simulink model "Copter_Plane_h2g_4_and_1_out"  (R2020a)
settings: Solver=ode1  StartTime=0.0  StopTime=1  FixedStep=dt  RelTol=1e-3
values from neighbouring files (symbols this model uses):
  center_WP = [40,100]*1e7    [Compter_Plane_inint_m_V10.m]    (also in Compter_Plane_inint_m_fs_form_V1031.m; Compter_Plane_inint_m_fs_form_V1032.m; Compter_Plane_inint_m_fs_form_V10321.m; Compter_Plane_inint_m_fs_form_V10321_4a1.m)
  Euler = [5/HD 5/HD 30/HD]    [Compter_Plane_inint_m_V10g.m]
  GRAVITY_MSS = 9.80665    [Compter_Plane_inint_m_V10.m]    (also in Compter_Plane_inint_m_V10g.m; Compter_Plane_inint_m_fs_form_V1031.m; Compter_Plane_inint_m_fs_form_V1032.m; Compter_Plane_inint_m_fs_form_V10321.m)
  gyro_x = 0    [Compter_Plane_inint_m_V10.m]    (also in Compter_Plane_inint_m_fs_form_V1031.m; Compter_Plane_inint_m_fs_form_V1032.m; Compter_Plane_inint_m_fs_form_V10321.m; Compter_Plane_inint_m_fs_form_V10321_4a1.m)
  gyro_y = 0/HD    (= 0)    [Compter_Plane_inint_m_V10.m]    (also in Compter_Plane_inint_m_fs_form_V1031.m; Compter_Plane_inint_m_fs_form_V1032.m; Compter_Plane_inint_m_fs_form_V10321.m; Compter_Plane_inint_m_fs_form_V10321_4a1.m)
  gyro_z = 0    [Compter_Plane_inint_m_V10.m]    (also in Compter_Plane_inint_m_fs_form_V1031.m; Compter_Plane_inint_m_fs_form_V1032.m; Compter_Plane_inint_m_fs_form_V10321.m; Compter_Plane_inint_m_fs_form_V10321_4a1.m)
  HD = 180/pi    (= 57.2957795131)    [Compter_Plane_inint_m_V10.m]    (also in Compter_Plane_inint_m_V10g.m; Compter_Plane_inint_m_fs_form_V1031.m; Compter_Plane_inint_m_fs_form_V1032.m; Compter_Plane_inint_m_fs_form_V10321.m)
  J = J_V10    [Compter_Plane_inint_m_V10.m]    (also in Compter_Plane_inint_m_V10g.m)
  Kd = Ku*Luy/Ldy    (= 18.9029535865)    [Compter_Plane_inint_m_V10.m]    (also in Compter_Plane_inint_m_fs_form_V1031.m; Compter_Plane_inint_m_fs_form_V1032.m; Compter_Plane_inint_m_fs_form_V10321.m; Compter_Plane_inint_m_fs_form_V10321_4a1.m)
  Ku = 32    [Compter_Plane_inint_m_V10.m]    (also in Compter_Plane_inint_m_fs_form_V1031.m; Compter_Plane_inint_m_fs_form_V1032.m; Compter_Plane_inint_m_fs_form_V10321.m; Compter_Plane_inint_m_fs_form_V10321_4a1.m)
  Ld = hypot(Ldx,Ldy)    [Compter_Plane_inint_m_V10.m]    (also in Compter_Plane_inint_m_fs_form_V1031.m; Compter_Plane_inint_m_fs_form_V1032.m; Compter_Plane_inint_m_fs_form_V10321.m; Compter_Plane_inint_m_fs_form_V10321_4a1.m)
  Ldx = 205/1000    (= 0.205)    [Compter_Plane_inint_m_V10.m]    (also in Compter_Plane_inint_m_fs_form_V1031.m; Compter_Plane_inint_m_fs_form_V1032.m; Compter_Plane_inint_m_fs_form_V10321.m; Compter_Plane_inint_m_fs_form_V10321_4a1.m)
  Ldy = 355.5/1000    (= 0.3555)    [Compter_Plane_inint_m_V10.m]    (also in Compter_Plane_inint_m_fs_form_V1031.m; Compter_Plane_inint_m_fs_form_V1032.m; Compter_Plane_inint_m_fs_form_V10321.m; Compter_Plane_inint_m_fs_form_V10321_4a1.m)
  Lu = hypot(Lux,Luy)    [Compter_Plane_inint_m_V10.m]    (also in Compter_Plane_inint_m_fs_form_V1031.m; Compter_Plane_inint_m_fs_form_V1032.m; Compter_Plane_inint_m_fs_form_V10321.m; Compter_Plane_inint_m_fs_form_V10321_4a1.m)
  Lux = 310/1000    (= 0.31)    [Compter_Plane_inint_m_V10.m]    (also in Compter_Plane_inint_m_fs_form_V1031.m; Compter_Plane_inint_m_fs_form_V1032.m; Compter_Plane_inint_m_fs_form_V10321.m; Compter_Plane_inint_m_fs_form_V10321_4a1.m)
  Luy = 210/1000    (= 0.21)    [Compter_Plane_inint_m_V10.m]    (also in Compter_Plane_inint_m_fs_form_V1031.m; Compter_Plane_inint_m_fs_form_V1032.m; Compter_Plane_inint_m_fs_form_V10321.m; Compter_Plane_inint_m_fs_form_V10321_4a1.m)
  m_kg = m_kg_V10    (= 26)    [Compter_Plane_inint_m_V10.m]    (also in Compter_Plane_inint_m_V10g.m; Compter_Plane_inint_m_fs_form_V1031.m = 5; Compter_Plane_inint_m_fs_form_V1032.m = 5; Compter_Plane_inint_m_fs_form_V10321.m = 5)
  pitch = -40/HD    (= -0.698131700798)    [Compter_Plane_inint_m_V10.m]    (also in Compter_Plane_inint_m_fs_form_V1031.m = 0; Compter_Plane_inint_m_fs_form_V1032.m = 0; Compter_Plane_inint_m_fs_form_V10321.m = 0; Compter_Plane_inint_m_fs_form_V10321_4a1.m = 0)
  pwm_max = 2000    [Compter_Plane_inint_m_V10.m]    (also in Compter_Plane_inint_m_fs_form_V1031.m; Compter_Plane_inint_m_fs_form_V1032.m; Compter_Plane_inint_m_fs_form_V10321.m; Compter_Plane_inint_m_fs_form_V10321_4a1.m)
  pwm_min = 1000    [Compter_Plane_inint_m_V10.m]    (also in Compter_Plane_inint_m_fs_form_V1031.m; Compter_Plane_inint_m_fs_form_V1032.m; Compter_Plane_inint_m_fs_form_V10321.m; Compter_Plane_inint_m_fs_form_V10321_4a1.m)
  Qd = 10    [Compter_Plane_inint_m_V10.m]    (also in Compter_Plane_inint_m_fs_form_V1031.m; Compter_Plane_inint_m_fs_form_V1032.m; Compter_Plane_inint_m_fs_form_V10321.m; Compter_Plane_inint_m_fs_form_V10321_4a1.m)
  Qu = asind(Kd*sind(Qd)*Ld/(Ku*Lu))    [Compter_Plane_inint_m_V10.m]    (also in Compter_Plane_inint_m_fs_form_V1031.m; Compter_Plane_inint_m_fs_form_V1032.m; Compter_Plane_inint_m_fs_form_V10321.m; Compter_Plane_inint_m_fs_form_V10321_4a1.m)
  roll = 10/HD    (= 0.174532925199)    [Compter_Plane_inint_m_V10.m]    (also in Compter_Plane_inint_m_fs_form_V1031.m = 0; Compter_Plane_inint_m_fs_form_V1032.m = 0; Compter_Plane_inint_m_fs_form_V10321.m = 0; Compter_Plane_inint_m_fs_form_V10321_4a1.m = 0)
  vel_desired = [0 0 0]    [Compter_Plane_inint_m_V10.m]    (also in Compter_Plane_inint_m_fs_form_V1031.m; Compter_Plane_inint_m_fs_form_V1032.m; Compter_Plane_inint_m_fs_form_V10321.m; Compter_Plane_inint_m_fs_form_V10321_4a1.m)
  yaw = 0    [Compter_Plane_inint_m_V10.m]    (also in Compter_Plane_inint_m_fs_form_V1031.m; Compter_Plane_inint_m_fs_form_V1032.m; Compter_Plane_inint_m_fs_form_V10321.m; Compter_Plane_inint_m_fs_form_V10321_4a1.m)
undefined symbols (not defined in the file or in its folder): Newton, QLd, QLdx, QLdy, QLu, QLux, QLuy, Raphson
libraries: shared6dofsys x3, sharedutil x1, simulink x1, aerolibasang x1
(part 1 of 3)
settings Model: xpc_rtwmakecfg_data=_xpcnblib_  PauseTimes=2  Creator=a4327  LastModifiedBy=a4327
settings DataIOCC: ReturnWorkspaceOutputs=off
settings OptimizationCC: DefaultParameterBehavior=Inlined  UseDivisionForNetSlopeComputation=on  GainParamInheritBuiltInType=on  UseFloatMulNetSlope=on  InlineInvariantSignals=on  PassReuseOutputArgsAs=Individual arguments  ZeroExternalMemoryAtStartup=off  ZeroInternalMemoryAtStartup=off  NoFixptDivByZeroProtection=on  EfficientFloat2IntCast=on  LifeSpan=1  OptimizeBlockOrder=speed  DifferentSizesBufferReuse=on  EfficientTunableParamExpr=on
settings DebuggingCC: ParameterTunabilityLossMsg=error  ArithmeticOperatorsInVariantConditions=warning
settings HardwareCC: ProdBitPerPointer=32  ProdBitPerSizeT=32  ProdBitPerPtrDiffT=32  ProdLargestAtomicFloat=None  ProdWordSize=32  ProdLongLongMode=on  ProdHWDeviceType=Custom Processor->Custom Processor
settings SFSimCC: MATLABDynamicMemAlloc=off  CustomCodeUndefinedFunction=UseInterfaceOnly
settings RTWCC: SystemTargetFile=ert.tlc  TemplateMakefile=ert_default_tmf  GenerateReport=on  IncludeHyperlinkInReport=on  LaunchReport=on  GenerateTraceInfo=on  GenerateTraceReport=on  GenerateTraceReportSl=on  GenerateTraceReportSf=on  GenerateTraceReportEml=on  GenerateCodeMetricsReport=on
settings CodeAppCC: ForceParamTrailComments=on  IgnoreCustomStorageClasses=off  OperatorAnnotations=on  SimulinkDataObjDesc=on  SFDataObjDesc=on  CustomSymbolStrGlobalVar=rt$N$M  CustomSymbolStrType=$N$M  CustomSymbolStrFcn=$N$M$F  CustomSymbolStrMacro=$N$M  InsertBlockDesc=on
settings ERTTargetCC: TargetLangStandard=C99 (ISO)  GenerateSampleERTMain=on  IncludeMdlTerminateFcn=off  CombineSignalStateStructs=on  MultiInstanceERTCode=on  CodeInterfacePackaging=Reusable function  SupportComplex=off  SupportNonInlinedSFcns=on  InlinedParameterPlacement=NonHierarchical  RootIOFormat=Structure reference  ERTCustomFileTemplate=example_file_process.tlc  ERTFilePackagingFormat=CompactWithDataFile

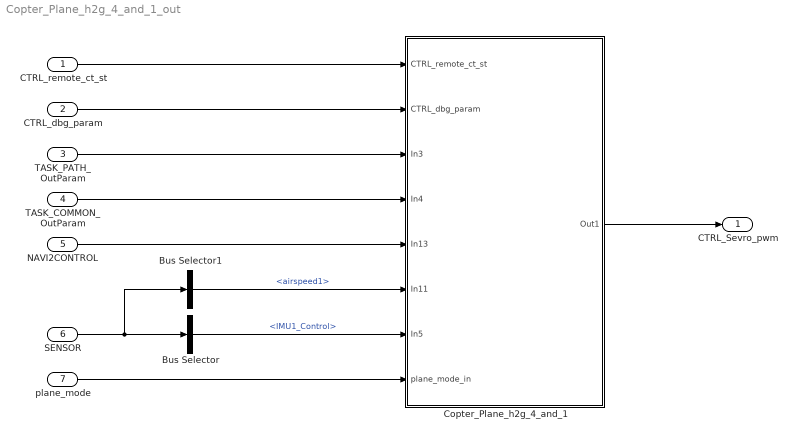
== system Copter_Plane_h2g_4_and_1_out ==
  CTRL_remote_ct_st : Inport  OutDataTypeStr=Bus: BUS_CTRL_remote_ct_st  BusOutputAsStruct=on
  CTRL_dbg_param : Inport  Port=2  OutDataTypeStr=Bus: BUS_CTRL_dbg_param  BusOutputAsStruct=on
  TASK_PATH_OutParam : Inport  Port=3  OutDataTypeStr=Bus: BUS_TASK_PATH_OutParam  BusOutputAsStruct=on
  TASK_COMMON_OutParam : Inport  Port=4  OutDataTypeStr=Bus: BUS_TASK_COMMON_OutParam  BusOutputAsStruct=on
  NAVI2CONTROL : Inport  Port=5  OutDataTypeStr=Bus: BUS_TO_CONTROL  BusOutputAsStruct=on
  SENSOR : Inport  Port=6  OutDataTypeStr=Bus: BUS_SENSOR
  plane_mode : Inport  Port=7  OutDataTypeStr=Enum: ENUM_plane_mode
  Bus Selector : BusSelector  OutputSignals=IMU1_Control
  Bus Selector1 : BusSelector  OutputSignals=airspeed1
  Copter_Plane_h2g_4_and_1 : Subsystem
  CTRL_Sevro_pwm : Outport  OutDataTypeStr=Bus: BUS_CTRL_Sevro_pwm
  wires:
  CTRL_dbg_param/1 -> Copter_Plane_h2g_4_and_1/2(CTRL_dbg_param)
  plane_mode/1 -> Copter_Plane_h2g_4_and_1/8(plane_mode_in)
  TASK_PATH_OutParam/1 -> Copter_Plane_h2g_4_and_1/3(In3)
  Bus Selector/1 -> Copter_Plane_h2g_4_and_1/7(In5)  "<IMU1_Control>"
  SENSOR/1 -> Bus Selector1/1, Bus Selector/1
  TASK_COMMON_OutParam/1 -> Copter_Plane_h2g_4_and_1/4(In4)
  NAVI2CONTROL/1 -> Copter_Plane_h2g_4_and_1/5(In13)
  Copter_Plane_h2g_4_and_1/1(Out1) -> CTRL_Sevro_pwm/1
  Bus Selector1/1 -> Copter_Plane_h2g_4_and_1/6(In11)  "<airspeed1>"
  CTRL_remote_ct_st/1 -> Copter_Plane_h2g_4_and_1/1(CTRL_remote_ct_st)
